simulink model "test_adc_ctrl"  (Simulink 7.4)
settings: Solver=ode45  StartTime=0.0  StopTime=100  RelTol=1e-3
libraries: xbsIndex_r4 x148, xps_library x36, isi_correlator_lib x19, dspsigops x16, casper_library x8
(part 1 of 2)
settings Model: Creator=wjm  LastModifiedBy=wjm
settings OptimizationCC: InitFltsAndDblsToZero=on

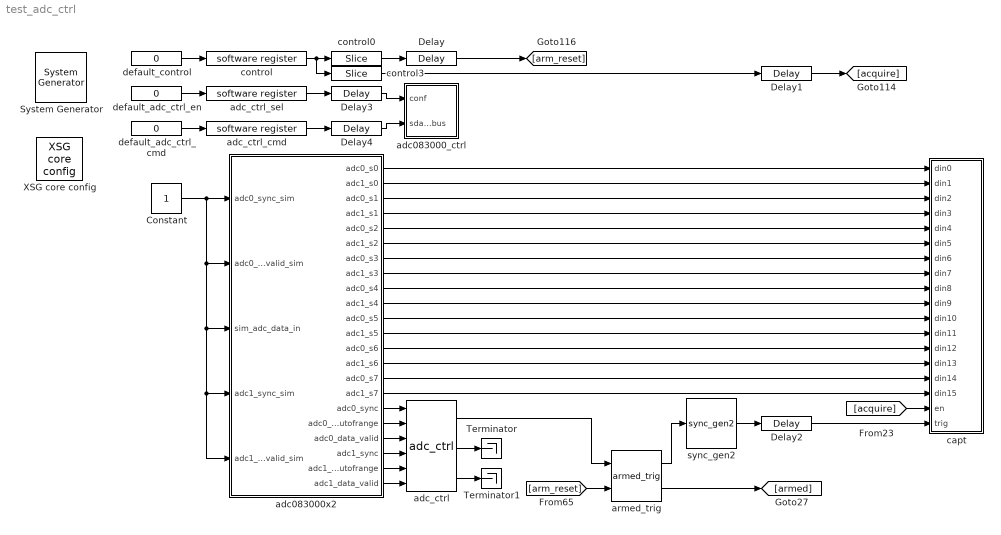
== system test_adc_ctrl ==
  " System Generator" : xbsIndex_r4/ System Generator  Tag=genX  SystemSampleTime=-1  xilinxfamily=virtex5  part=xc5vsx95t  speed=-1  package=ff1136  synthesis_tool=XST  clock_wrapper=Clock Enables  directory=./test_adc_ctrl/sysgen  testbench=off  simulink_period=1  sysclk_period=2.8571  dcm_input_clock_period=100  incr_netlist=off  trim_vbits=Everywhere in SubSystem  dbl_ovrd=According to Block Masks  core_generation=According to Block Masks  run_coregen=off  deprecated_control=off  eval_field=0  block_type=sysgen
      settings: block_version=10.1.3
  Constant : Constant  OutDataType=fixdt(1, 16)  OutScaling=2^0  SampleTime=1
  Delay : xbsIndex_r4/Delay  en=off  latency=5  dbl_ovrd=off  reg_retiming=on  block_type=delay
      settings: block_version=11.3
  Delay{1..4} (4 alike) : xbsIndex_r4/Delay  en=off  latency=3  dbl_ovrd=off  reg_retiming=on  block_type=delay
      settings: block_version=11.3
  Terminator : Terminator
  Terminator1 : Terminator
  XSG core config : xps_library/XSG core config  Tag=xps:xsg  SystemSampleTime=-1  hw_sys=ROACH:sx95t  ibob_linux=off  clk_src=adc0_clk  iBOB_clk_src=sys_clk  BEE2_ctrl_clk_src=sys_clk  BEE2_usr_clk_src=sys_clk  ROACH_clk_src=adc0_clk  CORR_clk_src=sys_clk  gpio_clk_io_group=iBOB:sma  gpio_clk_bit_index=0  clk_rate=350  sample_period=1  synthesis_tool=XST  mpc_type=powerpc440_ext
  adc083000_ctrl : Subsystem  Tag=xps:adc083000_ctrl  AncestorBlock=xps_library/ADCs/adc083000_ctrl  mask(adc083000_ctrl){}
      mask init:
      | adc083000_ctrl_mask;
  adc083000x2 : Subsystem  Tag=xps:adc083000x2  AncestorBlock=xps_library/adc083000x2  mask(adc_083000x2){use_adc0=on, use_adc1=on, demux_adc=off, clock_sync=on, verbose=off, using_ctrl=on, adc_clk_rate=1400, sample_period=1, bit_width=8}
      mask prompts: use_adc0 "Use ZD0K0?"; use_adc1 "Use ZDOK1?"; demux_adc "Demux ADCs by 2?"; clock_sync "Interleave 2 ADC boards?"; verbose "Verbose Block Creation?"; using_ctrl "Add ports for control registers?"; adc_clk_rate "ADC clock rate (MHz)"; sample_period "Sample Period"; bit_width "Output Bit Width"
      mask help:
      | The ADC block converts analog inputs to digital outputs.
      | Every clock cycle, the inputs are sampled and digitized to
      | 8 bit binary point numbers in the range of [-1, 1).
      |
      | Online block-specific documentation: http://casper.berkeley.edu/wiki/Adc083000
      mask init:
      | adc083000_mask;
      mask Help: eval('xlWeb([getenv(''MLIB_ROOT''), ''\doc\html\sys_adc\sys_adc.html''])')
  adc_ctrl : isi_correlator_lib/adc_ctrl  SystemSampleTime=-1
  adc_ctrl_cmd : xps_library/software register  Tag=xps:sw_reg  SystemSampleTime=-1  io_dir=From Processor  arith_type=Unsigned  bitwidth=32  bin_pt=0  sample_period=1  gw_name=test_adc_ctrl_adc_ctrl_cmd_user_data_out
  adc_ctrl_sel : xps_library/software register  Tag=xps:sw_reg  SystemSampleTime=-1  io_dir=From Processor  arith_type=Unsigned  bitwidth=32  bin_pt=0  sample_period=1  gw_name=test_adc_ctrl_adc_ctrl_sel_user_data_out
  armed_trig : isi_correlator_lib/armed_trig  SystemSampleTime=-1
  capt : Subsystem  AncestorBlock=isi_correlator_lib/capture  mask(capture){num_brams=16, addr_width=11, logic_latency=1, fanout_latency=1, cntr_latency=1, bram_latency=0}
      mask prompts: num_brams "Number of BRAMs:"; addr_width "Address width:"; logic_latency "Logic latency:"; fanout_latency "Fanout latency:"; cntr_latency "Counter latency:"; bram_latency "BRAM latency:"
      mask help: This block captures N data lines into N separate BRAMs.
      mask init:
      | capture_init(gcb, ...
      |     'num_brams', num_brams, ...
      |     'addr_width', addr_width, ...
      |     'logic_latency', logic_latency, ...
      |     'fanout_latency', fanout_latency, ...
      |     'cntr_latency', cntr_latency, ...
      |     'bram_latency', bram_latency);
  control : xps_library/software register  Tag=xps:sw_reg  SystemSampleTime=-1  io_dir=From Processor  arith_type=Unsigned  bitwidth=32  bin_pt=0  sample_period=1  gw_name=test_adc_ctrl_control_user_data_out
  control0 : xbsIndex_r4/Slice  nbits=1  boolean_output=on  mode=Lower Bit Location + Width  bit1=0  base1=MSB of Input  bit0=0  base0=LSB of Input  dbl_ovrd=off  block_type=slice
      settings: infoedit="Extracts a given range of bits from each input sample and presents it at the output.  The output type is ordinarily unsigned with binary point at zero, but can be Boolean when the slice is one bit wide.<P><P>Hardware notes: In hardware this block costs nothing."  block_version=10.1.3
  control3 : xbsIndex_r4/Slice  nbits=1  boolean_output=on  mode=Lower Bit Location + Width  bit1=0  base1=MSB of Input  bit0=3  base0=LSB of Input  dbl_ovrd=off  block_type=slice
      settings: infoedit="Extracts a given range of bits from each input sample and presents it at the output.  The output type is ordinarily unsigned with binary point at zero, but can be Boolean when the slice is one bit wide.<P><P>Hardware notes: In hardware this block costs nothing."  block_version=10.1.3
  default_adc_ctrl_cmd : Constant  Value=0  OutDataType=sfix(16)  OutScaling=2^0  SampleTime=1
  default_adc_ctrl_en : Constant  Value=0  OutDataType=sfix(16)  OutScaling=2^0  SampleTime=1
  default_control : Constant  Value=0  OutDataType=sfix(16)  OutScaling=2^0  SampleTime=1
  sync_gen2 : isi_correlator_lib/sync_gen2  SystemSampleTime=-1
  wires:
  adc083000x2/17(adc0_sync) -> adc_ctrl/1
  adc083000x2/18(adc0_outofrange) -> adc_ctrl/2
  adc083000x2/19(adc0_data_valid) -> adc_ctrl/3
  adc083000x2/20(adc1_sync) -> adc_ctrl/4
  adc083000x2/21(adc1_outofrange) -> adc_ctrl/5
  default_control/1 -> control/1
  control0/1 -> Delay/1
  control3/1 -> Delay1/1
  adc083000x2/22(adc1_data_valid) -> adc_ctrl/6
  adc_ctrl/2 -> Terminator/1
  adc_ctrl/3 -> Terminator1/1
  [arm_reset] -> armed_trig/2
  armed_trig/2 -> [armed]
  armed_trig/1 -> sync_gen2/1
  control/1 -> control0/1, control3/1
  Delay/1 -> [arm_reset]
  Delay1/1 -> [acquire]
  Constant/1 -> adc083000x2/1(adc0_sync_sim), adc083000x2/2(adc0_data_valid_sim), adc083000x2/3(sim_adc_data_in), adc083000x2/5(adc1_data_valid_sim), adc083000x2/4(adc1_sync_sim)
  adc_ctrl/1 -> armed_trig/1
  sync_gen2/1 -> Delay2/1
  adc_ctrl_sel/1 -> Delay3/1
  adc_ctrl_cmd/1 -> Delay4/1
  default_adc_ctrl_en/1 -> adc_ctrl_sel/1
  default_adc_ctrl_cmd/1 -> adc_ctrl_cmd/1
  Delay3/1 -> adc083000_ctrl/1(conf)
  Delay4/1 -> adc083000_ctrl/2(sdata_bus)
  adc083000x2/1(adc0_s0) -> capt/1(din0)
  adc083000x2/2(adc1_s0) -> capt/2(din1)
  adc083000x2/3(adc0_s1) -> capt/3(din2)
  adc083000x2/4(adc1_s1) -> capt/4(din3)
  adc083000x2/5(adc0_s2) -> capt/5(din4)
  adc083000x2/6(adc1_s2) -> capt/6(din5)
  adc083000x2/7(adc0_s3) -> capt/7(din6)
  adc083000x2/8(adc1_s3) -> capt/8(din7)
  adc083000x2/9(adc0_s4) -> capt/9(din8)
  adc083000x2/10(adc1_s4) -> capt/10(din9)
  adc083000x2/11(adc0_s5) -> capt/11(din10)
  adc083000x2/12(adc1_s5) -> capt/12(din11)
  adc083000x2/13(adc0_s6) -> capt/13(din12)
  adc083000x2/14(adc1_s6) -> capt/14(din13)
  adc083000x2/15(adc0_s7) -> capt/15(din14)
  adc083000x2/16(adc1_s7) -> capt/16(din15)
  [acquire] -> capt/17(en)
  Delay2/1 -> capt/18(trig)

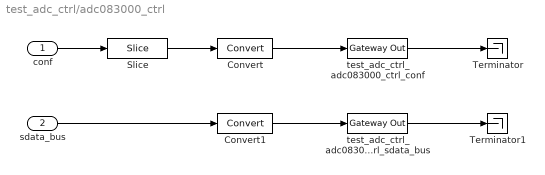
== system test_adc_ctrl/adc083000_ctrl ==
  conf : Inport  OutDataType=fixdt(1, 16)  OutScaling=2^0
  sdata_bus : Inport  Port=2  OutDataType=fixdt(1, 16)  OutScaling=2^0
  Convert : xbsIndex_r4/Convert  arith_type=Unsigned  n_bits=3  bin_pt=0  quantization=Truncate  overflow=Wrap  latency=2  dbl_ovrd=off  pipeline=off  block_type=convert
      settings: block_version=11.4
  Convert1 : xbsIndex_r4/Convert  arith_type=Unsigned  n_bits=32  bin_pt=0  quantization=Truncate  overflow=Wrap  latency=2  dbl_ovrd=off  pipeline=off  block_type=convert
      settings: block_version=11.4
  Slice : xbsIndex_r4/Slice  nbits=3  boolean_output=off  mode=Lower Bit Location + Width  bit1=0  base1=MSB of Input  bit0=0  base0=LSB of Input  dbl_ovrd=off  block_type=slice
  Terminator : Terminator
  Terminator1 : Terminator
  test_adc_ctrl_adc083000_ctrl_conf : xbsIndex_r4/Gateway Out  hdl_port=on  timing_constraint=None  locs_specified=off  LOCs={}  block_type=gatewayout
      settings: infoedit="Gateway out block.  Converts Xilinx fixed point inputs into ouputs of type Simulink integer, double, or fixed point.<br><br>Hardware notes:  In hardware these blocks become top level output ports or are discarded, depending on how they are configured."  block_version=11.4
  test_adc_ctrl_adc083000_ctrl_sdata_bus : xbsIndex_r4/Gateway Out  hdl_port=on  timing_constraint=None  locs_specified=off  LOCs={}  block_type=gatewayout
      settings: infoedit="Gateway out block.  Converts Xilinx fixed point inputs into ouputs of type Simulink integer, double, or fixed point.<br><br>Hardware notes:  In hardware these blocks become top level output ports or are discarded, depending on how they are configured."  block_version=11.4
  wires:
  sdata_bus/1 -> Convert1/1
  Convert/1 -> test_adc_ctrl_adc083000_ctrl_conf/1
  conf/1 -> Slice/1
  Slice/1 -> Convert/1
  Convert1/1 -> test_adc_ctrl_adc083000_ctrl_sdata_bus/1
  test_adc_ctrl_adc083000_ctrl_conf/1 -> Terminator/1
  test_adc_ctrl_adc083000_ctrl_sdata_bus/1 -> Terminator1/1

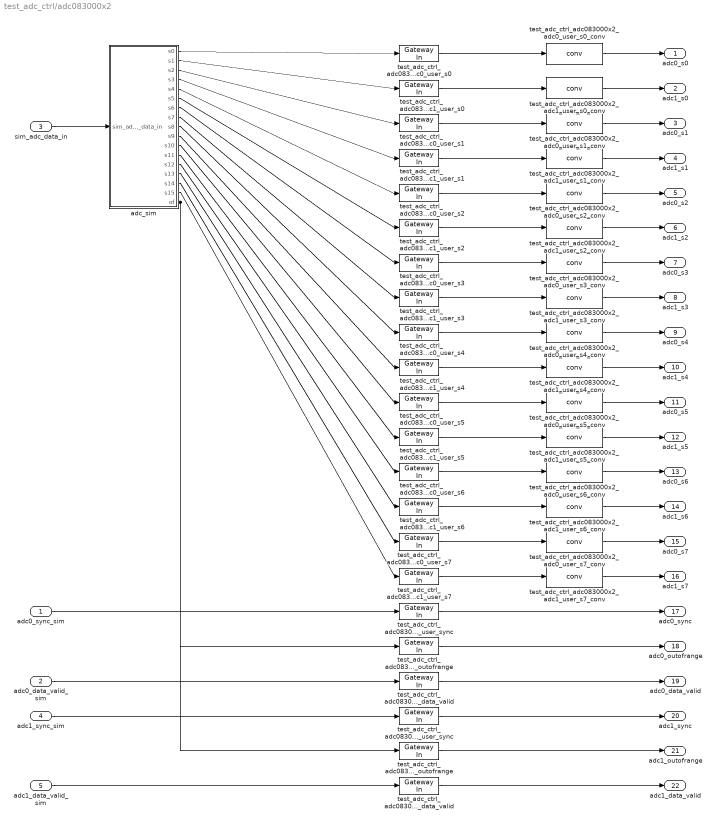
== system test_adc_ctrl/adc083000x2 ==
  adc0_sync_sim : Inport  OutDataType=sfix(16)  OutScaling=2^0
  adc0_data_valid_sim : Inport  Port=2  OutDataType=sfix(16)  OutScaling=2^0
  sim_adc_data_in : Inport  Port=3  OutDataType=fixdt(1, 16)  OutScaling=2^0
  adc1_sync_sim : Inport  Port=4  OutDataType=fixdt(1, 16)  OutScaling=2^0
  adc1_data_valid_sim : Inport  Port=5  OutDataType=fixdt(1, 16)  OutScaling=2^0
  adc_sim : Subsystem  AncestorBlock=xps_library/ADCs/adc_sim  mask(adc_sim){nStreams=16, bit_width=8}
      mask prompts: nStreams "Number of Output Streams"; bit_width "Sample Bit Width"
      mask help:
      | This block simulates the behavior of a demuxed ADC, which takes
      | as input a waveform and returns digital samples in parallel at
      | a slower rate.
      |
      | This block is used to simulate the behavior
      mask init:
      | adc_sim_init(gcb, ...
      |     'nStreams', nStreams, ...
      |     'bit_width', bit_width);
  test_adc_ctrl_adc083000x2_adc0_user_data_valid : xbsIndex_r4/Gateway In  arith_type=Unsigned  n_bits=1  bin_pt=0  quantization="Round  (unbiased: +/- Inf)"  overflow=Saturate  period=1  dbl_ovrd=off  timing_constraint=None  locs_specified=off  LOCs={}  hdl_port=on  block_type=gatewayin
      settings: infoedit="Gateway in block.  Converts inputs of type Simulink integer, double and fixed point to  Xilinx fixed point type.<br><br>Hardware notes:  In hardware these blocks become top level input ports."  block_version=11.4
  test_adc_ctrl_adc083000x2_adc0_user_outofrange : xbsIndex_r4/Gateway In  arith_type=Unsigned  n_bits=4  bin_pt=0  quantization="Round  (unbiased: +/- Inf)"  overflow=Saturate  period=1  dbl_ovrd=off  timing_constraint=None  locs_specified=off  LOCs={}  hdl_port=on  block_type=gatewayin
      settings: infoedit="Gateway in block.  Converts inputs of type Simulink integer, double and fixed point to  Xilinx fixed point type.<br><br>Hardware notes:  In hardware these blocks become top level input ports."  block_version=11.4
  test_adc_ctrl_adc083000x2_adc0_user_s{0..7} (8 alike) : xbsIndex_r4/Gateway In  arith_type=Unsigned  n_bits=8  bin_pt=0  quantization="Round  (unbiased: +/- Inf)"  overflow=Saturate  period=1  dbl_ovrd=off  timing_constraint=None  locs_specified=off  LOCs={}  hdl_port=on  block_type=gatewayin
      settings: infoedit="Gateway in block.  Converts inputs of type Simulink integer, double and fixed point to  Xilinx fixed point type.<br><br>Hardware notes:  In hardware these blocks become top level input ports."  block_version=11.4
  test_adc_ctrl_adc083000x2_adc0_user_s0_conv : xps_library/ADCs/conv  SystemSampleTime=-1  bit_width=8
  test_adc_ctrl_adc083000x2_adc0_user_s1_conv : xps_library/ADCs/conv  SystemSampleTime=-1  bit_width=8
  test_adc_ctrl_adc083000x2_adc0_user_s2_conv : xps_library/ADCs/conv  SystemSampleTime=-1  bit_width=8
  test_adc_ctrl_adc083000x2_adc0_user_s3_conv : xps_library/ADCs/conv  SystemSampleTime=-1  bit_width=8
  test_adc_ctrl_adc083000x2_adc0_user_s4_conv : xps_library/ADCs/conv  SystemSampleTime=-1  bit_width=8
  test_adc_ctrl_adc083000x2_adc0_user_s5_conv : xps_library/ADCs/conv  SystemSampleTime=-1  bit_width=8
  test_adc_ctrl_adc083000x2_adc0_user_s6_conv : xps_library/ADCs/conv  SystemSampleTime=-1  bit_width=8
  test_adc_ctrl_adc083000x2_adc0_user_s7_conv : xps_library/ADCs/conv  SystemSampleTime=-1  bit_width=8
  test_adc_ctrl_adc083000x2_adc0_user_sync : xbsIndex_r4/Gateway In  arith_type=Unsigned  n_bits=4  bin_pt=0  quantization="Round  (unbiased: +/- Inf)"  overflow=Saturate  period=1  dbl_ovrd=off  timing_constraint=None  locs_specified=off  LOCs={}  hdl_port=on  block_type=gatewayin
      settings: infoedit="Gateway in block.  Converts inputs of type Simulink integer, double and fixed point to  Xilinx fixed point type.<br><br>Hardware notes:  In hardware these blocks become top level input ports."  block_version=11.4
  test_adc_ctrl_adc083000x2_adc1_user_data_valid : xbsIndex_r4/Gateway In  arith_type=Unsigned  n_bits=1  bin_pt=0  quantization="Round  (unbiased: +/- Inf)"  overflow=Saturate  period=1  dbl_ovrd=off  timing_constraint=None  locs_specified=off  LOCs={}  hdl_port=on  block_type=gatewayin
      settings: infoedit="Gateway in block.  Converts inputs of type Simulink integer, double and fixed point to  Xilinx fixed point type.<br><br>Hardware notes:  In hardware these blocks become top level input ports."  block_version=11.4
  test_adc_ctrl_adc083000x2_adc1_user_outofrange : xbsIndex_r4/Gateway In  arith_type=Unsigned  n_bits=4  bin_pt=0  quantization="Round  (unbiased: +/- Inf)"  overflow=Saturate  period=1  dbl_ovrd=off  timing_constraint=None  locs_specified=off  LOCs={}  hdl_port=on  block_type=gatewayin
      settings: infoedit="Gateway in block.  Converts inputs of type Simulink integer, double and fixed point to  Xilinx fixed point type.<br><br>Hardware notes:  In hardware these blocks become top level input ports."  block_version=11.4
  test_adc_ctrl_adc083000x2_adc1_user_s{0..7} (8 alike) : xbsIndex_r4/Gateway In  arith_type=Unsigned  n_bits=8  bin_pt=0  quantization="Round  (unbiased: +/- Inf)"  overflow=Saturate  period=1  dbl_ovrd=off  timing_constraint=None  locs_specified=off  LOCs={}  hdl_port=on  block_type=gatewayin
      settings: infoedit="Gateway in block.  Converts inputs of type Simulink integer, double and fixed point to  Xilinx fixed point type.<br><br>Hardware notes:  In hardware these blocks become top level input ports."  block_version=11.4
  test_adc_ctrl_adc083000x2_adc1_user_s0_conv : xps_library/ADCs/conv  SystemSampleTime=-1  bit_width=8
  test_adc_ctrl_adc083000x2_adc1_user_s1_conv : xps_library/ADCs/conv  SystemSampleTime=-1  bit_width=8
  test_adc_ctrl_adc083000x2_adc1_user_s2_conv : xps_library/ADCs/conv  SystemSampleTime=-1  bit_width=8
  test_adc_ctrl_adc083000x2_adc1_user_s3_conv : xps_library/ADCs/conv  SystemSampleTime=-1  bit_width=8
  test_adc_ctrl_adc083000x2_adc1_user_s4_conv : xps_library/ADCs/conv  SystemSampleTime=-1  bit_width=8
  test_adc_ctrl_adc083000x2_adc1_user_s5_conv : xps_library/ADCs/conv  SystemSampleTime=-1  bit_width=8
  test_adc_ctrl_adc083000x2_adc1_user_s6_conv : xps_library/ADCs/conv  SystemSampleTime=-1  bit_width=8
  test_adc_ctrl_adc083000x2_adc1_user_s7_conv : xps_library/ADCs/conv  SystemSampleTime=-1  bit_width=8
  test_adc_ctrl_adc083000x2_adc1_user_sync : xbsIndex_r4/Gateway In  arith_type=Unsigned  n_bits=4  bin_pt=0  quantization="Round  (unbiased: +/- Inf)"  overflow=Saturate  period=1  dbl_ovrd=off  timing_constraint=None  locs_specified=off  LOCs={}  hdl_port=on  block_type=gatewayin
      settings: infoedit="Gateway in block.  Converts inputs of type Simulink integer, double and fixed point to  Xilinx fixed point type.<br><br>Hardware notes:  In hardware these blocks become top level input ports."  block_version=11.4
  adc0_s0 : Outport  OutDataType=fixdt(1, 16)  OutScaling=2^0
  adc1_s0 : Outport  Port=2  OutDataType=fixdt(1, 16)  OutScaling=2^0
  adc0_s1 : Outport  Port=3  OutDataType=fixdt(1, 16)  OutScaling=2^0
  adc1_s1 : Outport  Port=4  OutDataType=fixdt(1, 16)  OutScaling=2^0
  adc0_s2 : Outport  Port=5  OutDataType=fixdt(1, 16)  OutScaling=2^0
  adc1_s2 : Outport  Port=6  OutDataType=fixdt(1, 16)  OutScaling=2^0
  adc0_s3 : Outport  Port=7  OutDataType=fixdt(1, 16)  OutScaling=2^0
  adc1_s3 : Outport  Port=8  OutDataType=fixdt(1, 16)  OutScaling=2^0
  adc0_s4 : Outport  Port=9  OutDataType=fixdt(1, 16)  OutScaling=2^0
  adc1_s4 : Outport  Port=10  OutDataType=fixdt(1, 16)  OutScaling=2^0
  adc0_s5 : Outport  Port=11  OutDataType=fixdt(1, 16)  OutScaling=2^0
  adc1_s5 : Outport  Port=12  OutDataType=fixdt(1, 16)  OutScaling=2^0
  adc0_s6 : Outport  Port=13  OutDataType=fixdt(1, 16)  OutScaling=2^0
  adc1_s6 : Outport  Port=14  OutDataType=fixdt(1, 16)  OutScaling=2^0
  adc0_s7 : Outport  Port=15  OutDataType=fixdt(1, 16)  OutScaling=2^0
  adc1_s7 : Outport  Port=16  OutDataType=fixdt(1, 16)  OutScaling=2^0
  adc0_sync : Outport  Port=17  OutDataType=sfix(16)  OutScaling=2^0
  adc0_outofrange : Outport  Port=18  OutDataType=fixdt(1, 16)  OutScaling=2^0
  adc0_data_valid : Outport  Port=19  OutDataType=sfix(16)  OutScaling=2^0
  adc1_sync : Outport  Port=20  OutDataType=fixdt(1, 16)  OutScaling=2^0
  adc1_outofrange : Outport  Port=21  OutDataType=fixdt(1, 16)  OutScaling=2^0
  adc1_data_valid : Outport  Port=22  OutDataType=fixdt(1, 16)  OutScaling=2^0
  wires:
  sim_adc_data_in/1 -> adc_sim/1(sim_adc_data_in)
  adc_sim/1(s0) -> test_adc_ctrl_adc083000x2_adc0_user_s0/1
  test_adc_ctrl_adc083000x2_adc0_user_s0/1 -> test_adc_ctrl_adc083000x2_adc0_user_s0_conv/1
  test_adc_ctrl_adc083000x2_adc0_user_s0_conv/1 -> adc0_s0/1
  adc_sim/2(s1) -> test_adc_ctrl_adc083000x2_adc1_user_s0/1
  test_adc_ctrl_adc083000x2_adc1_user_s0/1 -> test_adc_ctrl_adc083000x2_adc1_user_s0_conv/1
  test_adc_ctrl_adc083000x2_adc1_user_s0_conv/1 -> adc1_s0/1
  adc_sim/3(s2) -> test_adc_ctrl_adc083000x2_adc0_user_s1/1
  test_adc_ctrl_adc083000x2_adc0_user_s1/1 -> test_adc_ctrl_adc083000x2_adc0_user_s1_conv/1
  test_adc_ctrl_adc083000x2_adc0_user_s1_conv/1 -> adc0_s1/1
  adc_sim/4(s3) -> test_adc_ctrl_adc083000x2_adc1_user_s1/1
  test_adc_ctrl_adc083000x2_adc1_user_s1/1 -> test_adc_ctrl_adc083000x2_adc1_user_s1_conv/1
  test_adc_ctrl_adc083000x2_adc1_user_s1_conv/1 -> adc1_s1/1
  adc_sim/5(s4) -> test_adc_ctrl_adc083000x2_adc0_user_s2/1
  test_adc_ctrl_adc083000x2_adc0_user_s2/1 -> test_adc_ctrl_adc083000x2_adc0_user_s2_conv/1
  test_adc_ctrl_adc083000x2_adc0_user_s2_conv/1 -> adc0_s2/1
  adc_sim/6(s5) -> test_adc_ctrl_adc083000x2_adc1_user_s2/1
  test_adc_ctrl_adc083000x2_adc1_user_s2/1 -> test_adc_ctrl_adc083000x2_adc1_user_s2_conv/1
  test_adc_ctrl_adc083000x2_adc1_user_s2_conv/1 -> adc1_s2/1
  adc_sim/7(s6) -> test_adc_ctrl_adc083000x2_adc0_user_s3/1
  test_adc_ctrl_adc083000x2_adc0_user_s3/1 -> test_adc_ctrl_adc083000x2_adc0_user_s3_conv/1
  test_adc_ctrl_adc083000x2_adc0_user_s3_conv/1 -> adc0_s3/1
  adc_sim/8(s7) -> test_adc_ctrl_adc083000x2_adc1_user_s3/1
  test_adc_ctrl_adc083000x2_adc1_user_s3/1 -> test_adc_ctrl_adc083000x2_adc1_user_s3_conv/1
  test_adc_ctrl_adc083000x2_adc1_user_s3_conv/1 -> adc1_s3/1
  adc_sim/9(s8) -> test_adc_ctrl_adc083000x2_adc0_user_s4/1
  test_adc_ctrl_adc083000x2_adc0_user_s4/1 -> test_adc_ctrl_adc083000x2_adc0_user_s4_conv/1
  test_adc_ctrl_adc083000x2_adc0_user_s4_conv/1 -> adc0_s4/1
  adc_sim/10(s9) -> test_adc_ctrl_adc083000x2_adc1_user_s4/1
  test_adc_ctrl_adc083000x2_adc1_user_s4/1 -> test_adc_ctrl_adc083000x2_adc1_user_s4_conv/1
  test_adc_ctrl_adc083000x2_adc1_user_s4_conv/1 -> adc1_s4/1
  adc_sim/11(s10) -> test_adc_ctrl_adc083000x2_adc0_user_s5/1
  test_adc_ctrl_adc083000x2_adc0_user_s5/1 -> test_adc_ctrl_adc083000x2_adc0_user_s5_conv/1
  test_adc_ctrl_adc083000x2_adc0_user_s5_conv/1 -> adc0_s5/1
  adc_sim/12(s11) -> test_adc_ctrl_adc083000x2_adc1_user_s5/1
  test_adc_ctrl_adc083000x2_adc1_user_s5/1 -> test_adc_ctrl_adc083000x2_adc1_user_s5_conv/1
  test_adc_ctrl_adc083000x2_adc1_user_s5_conv/1 -> adc1_s5/1
  adc_sim/13(s12) -> test_adc_ctrl_adc083000x2_adc0_user_s6/1
  test_adc_ctrl_adc083000x2_adc0_user_s6/1 -> test_adc_ctrl_adc083000x2_adc0_user_s6_conv/1
  test_adc_ctrl_adc083000x2_adc0_user_s6_conv/1 -> adc0_s6/1
  adc_sim/14(s13) -> test_adc_ctrl_adc083000x2_adc1_user_s6/1
  test_adc_ctrl_adc083000x2_adc1_user_s6/1 -> test_adc_ctrl_adc083000x2_adc1_user_s6_conv/1
  test_adc_ctrl_adc083000x2_adc1_user_s6_conv/1 -> adc1_s6/1
  adc_sim/15(s14) -> test_adc_ctrl_adc083000x2_adc0_user_s7/1
  test_adc_ctrl_adc083000x2_adc0_user_s7/1 -> test_adc_ctrl_adc083000x2_adc0_user_s7_conv/1
  test_adc_ctrl_adc083000x2_adc0_user_s7_conv/1 -> adc0_s7/1
  adc_sim/16(s15) -> test_adc_ctrl_adc083000x2_adc1_user_s7/1
  test_adc_ctrl_adc083000x2_adc1_user_s7/1 -> test_adc_ctrl_adc083000x2_adc1_user_s7_conv/1
  test_adc_ctrl_adc083000x2_adc1_user_s7_conv/1 -> adc1_s7/1
  adc0_sync_sim/1 -> test_adc_ctrl_adc083000x2_adc0_user_sync/1
  test_adc_ctrl_adc083000x2_adc0_user_sync/1 -> adc0_sync/1
  adc_sim/17(of) -> test_adc_ctrl_adc083000x2_adc0_user_outofrange/1, test_adc_ctrl_adc083000x2_adc1_user_outofrange/1
  test_adc_ctrl_adc083000x2_adc0_user_outofrange/1 -> adc0_outofrange/1
  adc0_data_valid_sim/1 -> test_adc_ctrl_adc083000x2_adc0_user_data_valid/1
  test_adc_ctrl_adc083000x2_adc0_user_data_valid/1 -> adc0_data_valid/1
  adc1_sync_sim/1 -> test_adc_ctrl_adc083000x2_adc1_user_sync/1
  test_adc_ctrl_adc083000x2_adc1_user_sync/1 -> adc1_sync/1
  test_adc_ctrl_adc083000x2_adc1_user_outofrange/1 -> adc1_outofrange/1
  adc1_data_valid_sim/1 -> test_adc_ctrl_adc083000x2_adc1_user_data_valid/1
  test_adc_ctrl_adc083000x2_adc1_user_data_valid/1 -> adc1_data_valid/1

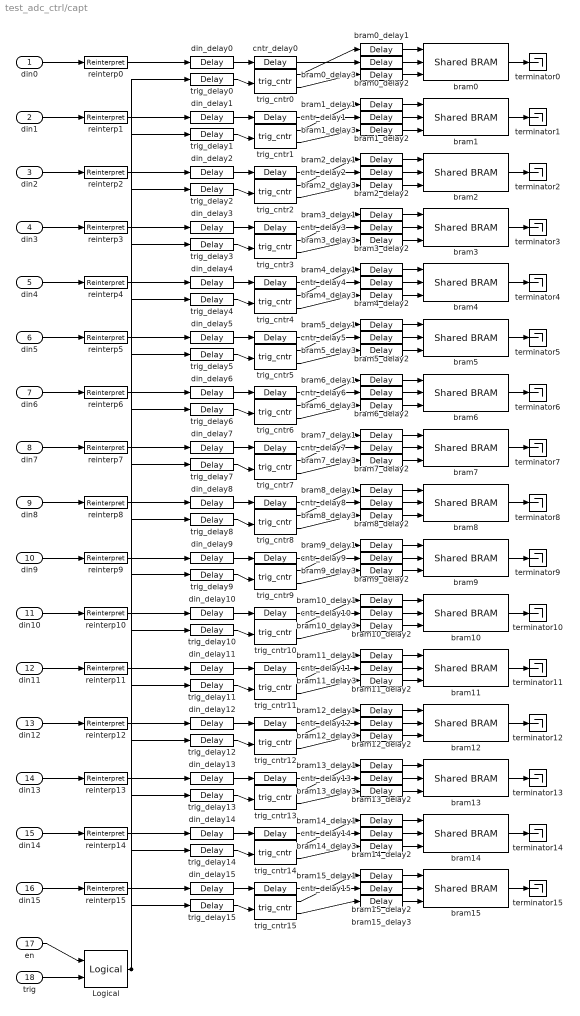
== system test_adc_ctrl/capt ==
  din0 : Inport
  din1 : Inport  Port=2
  din2 : Inport  Port=3
  din3 : Inport  Port=4
  din4 : Inport  Port=5
  din5 : Inport  Port=6
  din6 : Inport  Port=7
  din7 : Inport  Port=8
  din8 : Inport  Port=9
  din9 : Inport  Port=10
  din10 : Inport  Port=11
  din11 : Inport  Port=12
  din12 : Inport  Port=13
  din13 : Inport  Port=14
  din14 : Inport  Port=15
  din15 : Inport  Port=16
  en : Inport  Port=17
  trig : Inport  Port=18
  Logical : xbsIndex_r4/Logical  logical_function=AND  inputs=2  en=off  latency=logic_latency  precision=Full  arith_type=Unsigned  n_bits=16  bin_pt=0  align_bp=on  dbl_ovrd=off  block_type=logical
      settings: block_version=11.3
  bram{0..15} (16 alike) : xps_library/Shared BRAM  Tag=xps:bram  SystemSampleTime=-1  arith_type=Unsigned  addr_width=addr_width  data_width=32  data_bin_pt=0  init_vals=0  sample_rate=1
  bram0_delay1 : xbsIndex_r4/Delay  en=off  latency=bram_latency  dbl_ovrd=off  reg_retiming=on  block_type=delay
      settings: block_version=11.3
  bram0_delay2 : xbsIndex_r4/Delay  en=off  latency=bram_latency  dbl_ovrd=off  reg_retiming=on  block_type=delay
      settings: block_version=11.3
  bram0_delay3 : xbsIndex_r4/Delay  en=off  latency=bram_latency  dbl_ovrd=off  reg_retiming=on  block_type=delay
      settings: block_version=11.3
  bram10_delay1 : xbsIndex_r4/Delay  en=off  latency=bram_latency  dbl_ovrd=off  reg_retiming=on  block_type=delay
      settings: block_version=11.4
  bram10_delay2 : xbsIndex_r4/Delay  en=off  latency=bram_latency  dbl_ovrd=off  reg_retiming=on  block_type=delay
      settings: block_version=11.4
  bram10_delay3 : xbsIndex_r4/Delay  en=off  latency=bram_latency  dbl_ovrd=off  reg_retiming=on  block_type=delay
      settings: block_version=11.4
  bram11_delay1 : xbsIndex_r4/Delay  en=off  latency=bram_latency  dbl_ovrd=off  reg_retiming=on  block_type=delay
      settings: block_version=11.4
  bram11_delay2 : xbsIndex_r4/Delay  en=off  latency=bram_latency  dbl_ovrd=off  reg_retiming=on  block_type=delay
      settings: block_version=11.4
  bram11_delay3 : xbsIndex_r4/Delay  en=off  latency=bram_latency  dbl_ovrd=off  reg_retiming=on  block_type=delay
      settings: block_version=11.4
  bram12_delay1 : xbsIndex_r4/Delay  en=off  latency=bram_latency  dbl_ovrd=off  reg_retiming=on  block_type=delay
      settings: block_version=11.4
  bram12_delay2 : xbsIndex_r4/Delay  en=off  latency=bram_latency  dbl_ovrd=off  reg_retiming=on  block_type=delay
      settings: block_version=11.4
  bram12_delay3 : xbsIndex_r4/Delay  en=off  latency=bram_latency  dbl_ovrd=off  reg_retiming=on  block_type=delay
      settings: block_version=11.4
  bram13_delay1 : xbsIndex_r4/Delay  en=off  latency=bram_latency  dbl_ovrd=off  reg_retiming=on  block_type=delay
      settings: block_version=11.4
  bram13_delay2 : xbsIndex_r4/Delay  en=off  latency=bram_latency  dbl_ovrd=off  reg_retiming=on  block_type=delay
      settings: block_version=11.4
  bram13_delay3 : xbsIndex_r4/Delay  en=off  latency=bram_latency  dbl_ovrd=off  reg_retiming=on  block_type=delay
      settings: block_version=11.4
  bram14_delay1 : xbsIndex_r4/Delay  en=off  latency=bram_latency  dbl_ovrd=off  reg_retiming=on  block_type=delay
      settings: block_version=11.4
  bram14_delay2 : xbsIndex_r4/Delay  en=off  latency=bram_latency  dbl_ovrd=off  reg_retiming=on  block_type=delay
      settings: block_version=11.4
  bram14_delay3 : xbsIndex_r4/Delay  en=off  latency=bram_latency  dbl_ovrd=off  reg_retiming=on  block_type=delay
      settings: block_version=11.4
  bram15_delay1 : xbsIndex_r4/Delay  en=off  latency=bram_latency  dbl_ovrd=off  reg_retiming=on  block_type=delay
      settings: block_version=11.4
  bram15_delay2 : xbsIndex_r4/Delay  en=off  latency=bram_latency  dbl_ovrd=off  reg_retiming=on  block_type=delay
      settings: block_version=11.4
  bram15_delay3 : xbsIndex_r4/Delay  en=off  latency=bram_latency  dbl_ovrd=off  reg_retiming=on  block_type=delay
      settings: block_version=11.4
  bram1_delay1 : xbsIndex_r4/Delay  en=off  latency=bram_latency  dbl_ovrd=off  reg_retiming=on  block_type=delay
      settings: block_version=11.4
  bram1_delay2 : xbsIndex_r4/Delay  en=off  latency=bram_latency  dbl_ovrd=off  reg_retiming=on  block_type=delay
      settings: block_version=11.4
  bram1_delay3 : xbsIndex_r4/Delay  en=off  latency=bram_latency  dbl_ovrd=off  reg_retiming=on  block_type=delay
      settings: block_version=11.4
  bram2_delay1 : xbsIndex_r4/Delay  en=off  latency=bram_latency  dbl_ovrd=off  reg_retiming=on  block_type=delay
      settings: block_version=11.4
  bram2_delay2 : xbsIndex_r4/Delay  en=off  latency=bram_latency  dbl_ovrd=off  reg_retiming=on  block_type=delay
      settings: block_version=11.4
  bram2_delay3 : xbsIndex_r4/Delay  en=off  latency=bram_latency  dbl_ovrd=off  reg_retiming=on  block_type=delay
      settings: block_version=11.4
  bram3_delay1 : xbsIndex_r4/Delay  en=off  latency=bram_latency  dbl_ovrd=off  reg_retiming=on  block_type=delay
      settings: block_version=11.4
  bram3_delay2 : xbsIndex_r4/Delay  en=off  latency=bram_latency  dbl_ovrd=off  reg_retiming=on  block_type=delay
      settings: block_version=11.4
  bram3_delay3 : xbsIndex_r4/Delay  en=off  latency=bram_latency  dbl_ovrd=off  reg_retiming=on  block_type=delay
      settings: block_version=11.4
  bram4_delay1 : xbsIndex_r4/Delay  en=off  latency=bram_latency  dbl_ovrd=off  reg_retiming=on  block_type=delay
      settings: block_version=11.4
  bram4_delay2 : xbsIndex_r4/Delay  en=off  latency=bram_latency  dbl_ovrd=off  reg_retiming=on  block_type=delay
      settings: block_version=11.4
  bram4_delay3 : xbsIndex_r4/Delay  en=off  latency=bram_latency  dbl_ovrd=off  reg_retiming=on  block_type=delay
      settings: block_version=11.4
  bram5_delay1 : xbsIndex_r4/Delay  en=off  latency=bram_latency  dbl_ovrd=off  reg_retiming=on  block_type=delay
      settings: block_version=11.4
  bram5_delay2 : xbsIndex_r4/Delay  en=off  latency=bram_latency  dbl_ovrd=off  reg_retiming=on  block_type=delay
      settings: block_version=11.4
  bram5_delay3 : xbsIndex_r4/Delay  en=off  latency=bram_latency  dbl_ovrd=off  reg_retiming=on  block_type=delay
      settings: block_version=11.4
  bram6_delay1 : xbsIndex_r4/Delay  en=off  latency=bram_latency  dbl_ovrd=off  reg_retiming=on  block_type=delay
      settings: block_version=11.4
  bram6_delay2 : xbsIndex_r4/Delay  en=off  latency=bram_latency  dbl_ovrd=off  reg_retiming=on  block_type=delay
      settings: block_version=11.4
  bram6_delay3 : xbsIndex_r4/Delay  en=off  latency=bram_latency  dbl_ovrd=off  reg_retiming=on  block_type=delay
      settings: block_version=11.4
  bram7_delay1 : xbsIndex_r4/Delay  en=off  latency=bram_latency  dbl_ovrd=off  reg_retiming=on  block_type=delay
      settings: block_version=11.4
  bram7_delay2 : xbsIndex_r4/Delay  en=off  latency=bram_latency  dbl_ovrd=off  reg_retiming=on  block_type=delay
      settings: block_version=11.4
  bram7_delay3 : xbsIndex_r4/Delay  en=off  latency=bram_latency  dbl_ovrd=off  reg_retiming=on  block_type=delay
      settings: block_version=11.4
  bram8_delay1 : xbsIndex_r4/Delay  en=off  latency=bram_latency  dbl_ovrd=off  reg_retiming=on  block_type=delay
      settings: block_version=11.4
  bram8_delay2 : xbsIndex_r4/Delay  en=off  latency=bram_latency  dbl_ovrd=off  reg_retiming=on  block_type=delay
      settings: block_version=11.4
  bram8_delay3 : xbsIndex_r4/Delay  en=off  latency=bram_latency  dbl_ovrd=off  reg_retiming=on  block_type=delay
      settings: block_version=11.4
  bram9_delay1 : xbsIndex_r4/Delay  en=off  latency=bram_latency  dbl_ovrd=off  reg_retiming=on  block_type=delay
      settings: block_version=11.4
  bram9_delay2 : xbsIndex_r4/Delay  en=off  latency=bram_latency  dbl_ovrd=off  reg_retiming=on  block_type=delay
      settings: block_version=11.4
  bram9_delay3 : xbsIndex_r4/Delay  en=off  latency=bram_latency  dbl_ovrd=off  reg_retiming=on  block_type=delay
      settings: block_version=11.4
  cntr_delay{0..15} (16 alike) : xbsIndex_r4/Delay  en=off  latency=cntr_latency + 1  dbl_ovrd=off  reg_retiming=on  block_type=delay
      cntr_delay0 settings: block_version=11.3
      cntr_delay1 settings: block_version=11.4
      cntr_delay10 settings: block_version=11.4
      cntr_delay11 settings: block_version=11.4
      cntr_delay12 settings: block_version=11.4
      cntr_delay13 settings: block_version=11.4
      cntr_delay14 settings: block_version=11.4
      cntr_delay15 settings: block_version=11.4
      cntr_delay2 settings: block_version=11.4
      cntr_delay3 settings: block_version=11.4
      cntr_delay4 settings: block_version=11.4
      cntr_delay5 settings: block_version=11.4
      cntr_delay6 settings: block_version=11.4
      cntr_delay7 settings: block_version=11.4
      cntr_delay8 settings: block_version=11.4
      cntr_delay9 settings: block_version=11.4
  din_delay{0..15} (16 alike) : xbsIndex_r4/Delay  en=off  latency=logic_latency + fanout_latency  dbl_ovrd=off  reg_retiming=on  block_type=delay
      din_delay0 settings: block_version=11.3
      din_delay1 settings: block_version=11.4
      din_delay10 settings: block_version=11.4
      din_delay11 settings: block_version=11.4
      din_delay12 settings: block_version=11.4
      din_delay13 settings: block_version=11.4
      din_delay14 settings: block_version=11.4
      din_delay15 settings: block_version=11.4
      din_delay2 settings: block_version=11.4
      din_delay3 settings: block_version=11.4
      din_delay4 settings: block_version=11.4
      din_delay5 settings: block_version=11.4
      din_delay6 settings: block_version=11.4
      din_delay7 settings: block_version=11.4
      din_delay8 settings: block_version=11.4
      din_delay9 settings: block_version=11.4
  reinterp{0..15} (16 alike) : xbsIndex_r4/Reinterpret  force_arith_type=on  arith_type=Unsigned  force_bin_pt=on  bin_pt=0  block_type=reinterpret
      reinterp0 settings: infoedit="Changes signal type without altering the binary representation.   You can changed the signal between signed and unsigned, and relocate the binary point.<br><br>Hardware notes: In hardware this block costs nothing.<br><br>Example:  Suppose the input is 6 bits wide, signed, with 2 fractional bits, and the output is forced to unsigned with 0 fractional bits.  Then an input of -2.0 (1110.00 in binary 2's complement) becomes an output of 56 (111000 in binary)."  block_version=11.3
      reinterp1 settings: infoedit="Changes signal type without altering the binary representation.   You can changed the signal between signed and unsigned, and relocate the binary point.<br><br>Hardware notes: In hardware this block costs nothing.<br><br>Example:  Suppose the input is 6 bits wide, signed, with 2 fractional bits, and the output is forced to unsigned with 0 fractional bits.  Then an input of -2.0 (1110.00 in binary 2's complement) becomes an output of 56 (111000 in binary)."
      reinterp10 settings: infoedit="Changes signal type without altering the binary representation.   You can changed the signal between signed and unsigned, and relocate the binary point.<br><br>Hardware notes: In hardware this block costs nothing.<br><br>Example:  Suppose the input is 6 bits wide, signed, with 2 fractional bits, and the output is forced to unsigned with 0 fractional bits.  Then an input of -2.0 (1110.00 in binary 2's complement) becomes an output of 56 (111000 in binary)."
      reinterp11 settings: infoedit="Changes signal type without altering the binary representation.   You can changed the signal between signed and unsigned, and relocate the binary point.<br><br>Hardware notes: In hardware this block costs nothing.<br><br>Example:  Suppose the input is 6 bits wide, signed, with 2 fractional bits, and the output is forced to unsigned with 0 fractional bits.  Then an input of -2.0 (1110.00 in binary 2's complement) becomes an output of 56 (111000 in binary)."
      reinterp12 settings: infoedit="Changes signal type without altering the binary representation.   You can changed the signal between signed and unsigned, and relocate the binary point.<br><br>Hardware notes: In hardware this block costs nothing.<br><br>Example:  Suppose the input is 6 bits wide, signed, with 2 fractional bits, and the output is forced to unsigned with 0 fractional bits.  Then an input of -2.0 (1110.00 in binary 2's complement) becomes an output of 56 (111000 in binary)."
      reinterp13 settings: infoedit="Changes signal type without altering the binary representation.   You can changed the signal between signed and unsigned, and relocate the binary point.<br><br>Hardware notes: In hardware this block costs nothing.<br><br>Example:  Suppose the input is 6 bits wide, signed, with 2 fractional bits, and the output is forced to unsigned with 0 fractional bits.  Then an input of -2.0 (1110.00 in binary 2's complement) becomes an output of 56 (111000 in binary)."
      reinterp14 settings: infoedit="Changes signal type without altering the binary representation.   You can changed the signal between signed and unsigned, and relocate the binary point.<br><br>Hardware notes: In hardware this block costs nothing.<br><br>Example:  Suppose the input is 6 bits wide, signed, with 2 fractional bits, and the output is forced to unsigned with 0 fractional bits.  Then an input of -2.0 (1110.00 in binary 2's complement) becomes an output of 56 (111000 in binary)."
      reinterp15 settings: infoedit="Changes signal type without altering the binary representation.   You can changed the signal between signed and unsigned, and relocate the binary point.<br><br>Hardware notes: In hardware this block costs nothing.<br><br>Example:  Suppose the input is 6 bits wide, signed, with 2 fractional bits, and the output is forced to unsigned with 0 fractional bits.  Then an input of -2.0 (1110.00 in binary 2's complement) becomes an output of 56 (111000 in binary)."
      reinterp2 settings: infoedit="Changes signal type without altering the binary representation.   You can changed the signal between signed and unsigned, and relocate the binary point.<br><br>Hardware notes: In hardware this block costs nothing.<br><br>Example:  Suppose the input is 6 bits wide, signed, with 2 fractional bits, and the output is forced to unsigned with 0 fractional bits.  Then an input of -2.0 (1110.00 in binary 2's complement) becomes an output of 56 (111000 in binary)."
      reinterp3 settings: infoedit="Changes signal type without altering the binary representation.   You can changed the signal between signed and unsigned, and relocate the binary point.<br><br>Hardware notes: In hardware this block costs nothing.<br><br>Example:  Suppose the input is 6 bits wide, signed, with 2 fractional bits, and the output is forced to unsigned with 0 fractional bits.  Then an input of -2.0 (1110.00 in binary 2's complement) becomes an output of 56 (111000 in binary)."
      reinterp4 settings: infoedit="Changes signal type without altering the binary representation.   You can changed the signal between signed and unsigned, and relocate the binary point.<br><br>Hardware notes: In hardware this block costs nothing.<br><br>Example:  Suppose the input is 6 bits wide, signed, with 2 fractional bits, and the output is forced to unsigned with 0 fractional bits.  Then an input of -2.0 (1110.00 in binary 2's complement) becomes an output of 56 (111000 in binary)."
      reinterp5 settings: infoedit="Changes signal type without altering the binary representation.   You can changed the signal between signed and unsigned, and relocate the binary point.<br><br>Hardware notes: In hardware this block costs nothing.<br><br>Example:  Suppose the input is 6 bits wide, signed, with 2 fractional bits, and the output is forced to unsigned with 0 fractional bits.  Then an input of -2.0 (1110.00 in binary 2's complement) becomes an output of 56 (111000 in binary)."
      reinterp6 settings: infoedit="Changes signal type without altering the binary representation.   You can changed the signal between signed and unsigned, and relocate the binary point.<br><br>Hardware notes: In hardware this block costs nothing.<br><br>Example:  Suppose the input is 6 bits wide, signed, with 2 fractional bits, and the output is forced to unsigned with 0 fractional bits.  Then an input of -2.0 (1110.00 in binary 2's complement) becomes an output of 56 (111000 in binary)."
      reinterp7 settings: infoedit="Changes signal type without altering the binary representation.   You can changed the signal between signed and unsigned, and relocate the binary point.<br><br>Hardware notes: In hardware this block costs nothing.<br><br>Example:  Suppose the input is 6 bits wide, signed, with 2 fractional bits, and the output is forced to unsigned with 0 fractional bits.  Then an input of -2.0 (1110.00 in binary 2's complement) becomes an output of 56 (111000 in binary)."
      reinterp8 settings: infoedit="Changes signal type without altering the binary representation.   You can changed the signal between signed and unsigned, and relocate the binary point.<br><br>Hardware notes: In hardware this block costs nothing.<br><br>Example:  Suppose the input is 6 bits wide, signed, with 2 fractional bits, and the output is forced to unsigned with 0 fractional bits.  Then an input of -2.0 (1110.00 in binary 2's complement) becomes an output of 56 (111000 in binary)."
      reinterp9 settings: infoedit="Changes signal type without altering the binary representation.   You can changed the signal between signed and unsigned, and relocate the binary point.<br><br>Hardware notes: In hardware this block costs nothing.<br><br>Example:  Suppose the input is 6 bits wide, signed, with 2 fractional bits, and the output is forced to unsigned with 0 fractional bits.  Then an input of -2.0 (1110.00 in binary 2's complement) becomes an output of 56 (111000 in binary)."
  terminator{0..15} (16 alike) : Terminator
  trig_cntr{0..15} (16 alike) : isi_correlator_lib/trig_cntr  SystemSampleTime=-1  bitwidth=addr_width  latency=cntr_latency
  trig_delay{0..15} (16 alike) : xbsIndex_r4/Delay  en=off  latency=fanout_latency  dbl_ovrd=off  reg_retiming=on  block_type=delay
      trig_delay0 settings: block_version=11.3
      trig_delay1 settings: block_version=11.4
      trig_delay10 settings: block_version=11.4
      trig_delay11 settings: block_version=11.4
      trig_delay12 settings: block_version=11.4
      trig_delay13 settings: block_version=11.4
      trig_delay14 settings: block_version=11.4
      trig_delay15 settings: block_version=11.4
      trig_delay2 settings: block_version=11.4
      trig_delay3 settings: block_version=11.4
      trig_delay4 settings: block_version=11.4
      trig_delay5 settings: block_version=11.4
      trig_delay6 settings: block_version=11.4
      trig_delay7 settings: block_version=11.4
      trig_delay8 settings: block_version=11.4
      trig_delay9 settings: block_version=11.4
  wires:
  bram0_delay1/1 -> bram0/1
  bram0_delay3/1 -> bram0/3
  din0/1 -> reinterp0/1
  reinterp0/1 -> din_delay0/1
  din_delay0/1 -> cntr_delay0/1
  cntr_delay0/1 -> bram0_delay2/1
  bram0_delay2/1 -> bram0/2
  bram0/1 -> terminator0/1
  trig_delay0/1 -> trig_cntr0/1
  trig_cntr0/1 -> bram0_delay1/1
  trig_cntr0/2 -> bram0_delay3/1
  bram1_delay1/1 -> bram1/1
  bram1_delay3/1 -> bram1/3
  din1/1 -> reinterp1/1
  reinterp1/1 -> din_delay1/1
  din_delay1/1 -> cntr_delay1/1
  cntr_delay1/1 -> bram1_delay2/1
  bram1_delay2/1 -> bram1/2
  bram1/1 -> terminator1/1
  trig_delay1/1 -> trig_cntr1/1
  trig_cntr1/1 -> bram1_delay1/1
  trig_cntr1/2 -> bram1_delay3/1
  bram2_delay1/1 -> bram2/1
  bram2_delay3/1 -> bram2/3
  din2/1 -> reinterp2/1
  reinterp2/1 -> din_delay2/1
  din_delay2/1 -> cntr_delay2/1
  cntr_delay2/1 -> bram2_delay2/1
  bram2_delay2/1 -> bram2/2
  bram2/1 -> terminator2/1
  trig_delay2/1 -> trig_cntr2/1
  trig_cntr2/1 -> bram2_delay1/1
  trig_cntr2/2 -> bram2_delay3/1
  bram3_delay1/1 -> bram3/1
  bram3_delay3/1 -> bram3/3
  din3/1 -> reinterp3/1
  reinterp3/1 -> din_delay3/1
  din_delay3/1 -> cntr_delay3/1
  cntr_delay3/1 -> bram3_delay2/1
  bram3_delay2/1 -> bram3/2
  bram3/1 -> terminator3/1
  trig_delay3/1 -> trig_cntr3/1
  trig_cntr3/1 -> bram3_delay1/1
  trig_cntr3/2 -> bram3_delay3/1
  bram4_delay1/1 -> bram4/1
  bram4_delay3/1 -> bram4/3
  din4/1 -> reinterp4/1
  reinterp4/1 -> din_delay4/1
  din_delay4/1 -> cntr_delay4/1
  cntr_delay4/1 -> bram4_delay2/1
  bram4_delay2/1 -> bram4/2
  bram4/1 -> terminator4/1
  trig_delay4/1 -> trig_cntr4/1
  trig_cntr4/1 -> bram4_delay1/1
  trig_cntr4/2 -> bram4_delay3/1
  bram5_delay1/1 -> bram5/1
  bram5_delay3/1 -> bram5/3
  din5/1 -> reinterp5/1
  reinterp5/1 -> din_delay5/1
  din_delay5/1 -> cntr_delay5/1
  cntr_delay5/1 -> bram5_delay2/1
  bram5_delay2/1 -> bram5/2
  bram5/1 -> terminator5/1
  trig_delay5/1 -> trig_cntr5/1
  trig_cntr5/1 -> bram5_delay1/1
  trig_cntr5/2 -> bram5_delay3/1
  bram6_delay1/1 -> bram6/1
  bram6_delay3/1 -> bram6/3
  din6/1 -> reinterp6/1
  reinterp6/1 -> din_delay6/1
  din_delay6/1 -> cntr_delay6/1
  cntr_delay6/1 -> bram6_delay2/1
  bram6_delay2/1 -> bram6/2
  bram6/1 -> terminator6/1
  trig_delay6/1 -> trig_cntr6/1
  trig_cntr6/1 -> bram6_delay1/1
  trig_cntr6/2 -> bram6_delay3/1
  bram7_delay1/1 -> bram7/1
  bram7_delay3/1 -> bram7/3
  din7/1 -> reinterp7/1
  reinterp7/1 -> din_delay7/1
  din_delay7/1 -> cntr_delay7/1
  cntr_delay7/1 -> bram7_delay2/1
  bram7_delay2/1 -> bram7/2
  bram7/1 -> terminator7/1
  trig_delay7/1 -> trig_cntr7/1
  trig_cntr7/1 -> bram7_delay1/1
  trig_cntr7/2 -> bram7_delay3/1
  bram8_delay1/1 -> bram8/1
  bram8_delay3/1 -> bram8/3
  din8/1 -> reinterp8/1
  reinterp8/1 -> din_delay8/1
  din_delay8/1 -> cntr_delay8/1
  cntr_delay8/1 -> bram8_delay2/1
  bram8_delay2/1 -> bram8/2
  bram8/1 -> terminator8/1
  trig_delay8/1 -> trig_cntr8/1
  trig_cntr8/1 -> bram8_delay1/1
  trig_cntr8/2 -> bram8_delay3/1
  bram9_delay1/1 -> bram9/1
  bram9_delay3/1 -> bram9/3
  din9/1 -> reinterp9/1
  reinterp9/1 -> din_delay9/1
  din_delay9/1 -> cntr_delay9/1
  cntr_delay9/1 -> bram9_delay2/1
  bram9_delay2/1 -> bram9/2
  bram9/1 -> terminator9/1
  trig_delay9/1 -> trig_cntr9/1
  trig_cntr9/1 -> bram9_delay1/1
  trig_cntr9/2 -> bram9_delay3/1
  bram10_delay1/1 -> bram10/1
  bram10_delay3/1 -> bram10/3
  din10/1 -> reinterp10/1
  reinterp10/1 -> din_delay10/1
  din_delay10/1 -> cntr_delay10/1
  cntr_delay10/1 -> bram10_delay2/1
  bram10_delay2/1 -> bram10/2
  bram10/1 -> terminator10/1
  trig_delay10/1 -> trig_cntr10/1
  trig_cntr10/1 -> bram10_delay1/1
  trig_cntr10/2 -> bram10_delay3/1
  bram11_delay1/1 -> bram11/1
  bram11_delay3/1 -> bram11/3
  din11/1 -> reinterp11/1
  reinterp11/1 -> din_delay11/1
  din_delay11/1 -> cntr_delay11/1
  cntr_delay11/1 -> bram11_delay2/1
  bram11_delay2/1 -> bram11/2
  bram11/1 -> terminator11/1
  trig_delay11/1 -> trig_cntr11/1
  trig_cntr11/1 -> bram11_delay1/1
  trig_cntr11/2 -> bram11_delay3/1
  bram12_delay1/1 -> bram12/1
  bram12_delay3/1 -> bram12/3
  din12/1 -> reinterp12/1
  reinterp12/1 -> din_delay12/1
  din_delay12/1 -> cntr_delay12/1
  cntr_delay12/1 -> bram12_delay2/1
  bram12_delay2/1 -> bram12/2
  bram12/1 -> terminator12/1
  trig_delay12/1 -> trig_cntr12/1
  trig_cntr12/1 -> bram12_delay1/1
  trig_cntr12/2 -> bram12_delay3/1
  bram13_delay1/1 -> bram13/1
  bram13_delay3/1 -> bram13/3
  din13/1 -> reinterp13/1
  reinterp13/1 -> din_delay13/1
  din_delay13/1 -> cntr_delay13/1
  cntr_delay13/1 -> bram13_delay2/1
  bram13_delay2/1 -> bram13/2
  bram13/1 -> terminator13/1
  trig_delay13/1 -> trig_cntr13/1
  trig_cntr13/1 -> bram13_delay1/1
  trig_cntr13/2 -> bram13_delay3/1
  bram14_delay1/1 -> bram14/1
  bram14_delay3/1 -> bram14/3
  din14/1 -> reinterp14/1
  reinterp14/1 -> din_delay14/1
  din_delay14/1 -> cntr_delay14/1
  cntr_delay14/1 -> bram14_delay2/1
  bram14_delay2/1 -> bram14/2
  bram14/1 -> terminator14/1
  trig_delay14/1 -> trig_cntr14/1
  trig_cntr14/1 -> bram14_delay1/1
  trig_cntr14/2 -> bram14_delay3/1
  bram15_delay1/1 -> bram15/1
  bram15_delay3/1 -> bram15/3
  din15/1 -> reinterp15/1
  reinterp15/1 -> din_delay15/1
  din_delay15/1 -> cntr_delay15/1
  cntr_delay15/1 -> bram15_delay2/1
  bram15_delay2/1 -> bram15/2
  bram15/1 -> terminator15/1
  trig_delay15/1 -> trig_cntr15/1
  trig_cntr15/1 -> bram15_delay1/1
  trig_cntr15/2 -> bram15_delay3/1
  en/1 -> Logical/1
  trig/1 -> Logical/2
  Logical/1 -> trig_delay0/1, trig_delay1/1, trig_delay2/1, trig_delay3/1, trig_delay4/1, trig_delay5/1, trig_delay6/1, trig_delay7/1, trig_delay8/1, trig_delay9/1, trig_delay10/1, trig_delay11/1, trig_delay12/1, trig_delay13/1, trig_delay14/1, trig_delay15/1
